simulink model "use_test"  (R2013a)
settings: Solver=ode45  StartTime=0.0  StopTime=1  RelTol=1e-3
settings Model: Creator=Nathan  LastModifiedBy=Nathan

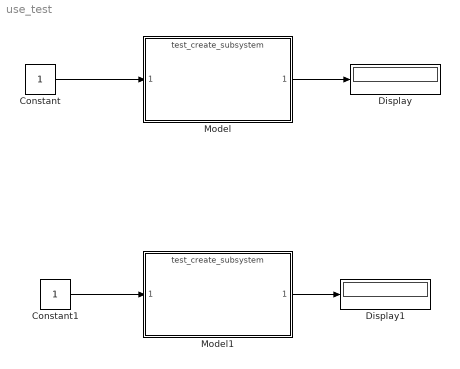
== system use_test ==
  Constant : Constant
  Constant1 : Constant
  Display : Display
  Display1 : Display
  Model : ModelReference  ModelNameDialog=test_create_subsystem.slx  SimulationMode=Normal  ModelReferenceVersion=1.14  CopyOfModelName=test_create_subsystem.slx  DefaultDataLogging=on
  Model1 : ModelReference  ModelNameDialog=test_create_subsystem.slx  SimulationMode=Normal  ModelReferenceVersion=1.14  CopyOfModelName=test_create_subsystem.slx  DefaultDataLogging=on
  wires:
  Constant/1 -> Model/1
  Model/1 -> Display/1
  Constant1/1 -> Model1/1
  Model1/1 -> Display1/1
